simulink model "rendezvous_optimization_ALO"  (R2023a)
settings: Solver=VariableStepAuto  StartTime=0.0  StopTime=600  RelTol=1e-3
undefined symbols (not defined in the file): Ax, Ax_i, Ay, Ay_i, Az, Bx, Bx_i, By, By_i, Bz, Cx, Cx_i, Cy, Cy_i, Cz, IC_x_init, IC_y_init, juliandate, m0, mDot, OC_x_init, OC_y_init, OC_z_init, omega_T, Ve
(part 2 of 2)

== matlab function rendezvous_optimization_ALO/Deputy Spacecraft/Guidance and Control/Control/Translational Controller/MATLAB Function3 ==
  data: rc_N input; Fb_Hill output; vc_N input; Fb_ICRF input
function Fb_Hill = convertForceICRFtoHill(rc_N, vc_N, Fb_ICRF)
%#codegen
% Converts a force vector from ICRF frame to Hill frame
%
% Inputs:
%   rc_N     - Chief inertial position (3x1)
%   vc_N     - Chief inertial velocity (3x1)
%   Fb_ICRF  - Force vector in ICRF frame (3x1)
%
% Output:
%   Fb_Hill  - Force vector in Hill frame (3x1)

% Normalize radial (x) direction
ir = rc_N / norm(rc_N);

% Compute angular momentum vector and normalize (z-direction)
h = cross(rc_N, vc_N);
ih = h / norm(h);

% Compute along-track (y) direction
itheta = cross(ih, ir);

% Construct rotation matrix: Hill to ICRF
R_hill_to_icrf = [ir, itheta, ih];

% To convert from ICRF to Hill: transpose (inverse of rotation matrix)
R_icrf_to_hill = R_hill_to_icrf';

% Rotate force vector into Hill frame
Fb_Hill = R_icrf_to_hill * Fb_ICRF;

end

== matlab function rendezvous_optimization_ALO/Deputy Spacecraft/Guidance and Control/Control/Translational Controller/Outer Controller-x/Controller-1/MATLAB Function ==
  settings: updateMethod=DISCRETE
  data: bestKi output; bestKp output; bestKd output; error input
function [bestKi,bestKp,bestKd] = antlion(error)
% antlion  Tune PID gains [Kp,Ki,Kd] via Ant Lion Optimizer
%
%   sys  = your state‐space or transfer‐function plant
%   [bestKp,bestKi,bestKd] = antlion(sys)

  %% ALO parameters
  nAnt     = 20;          
  Max_iter = 100;
  dim = 3;
  lb       = [0   0   0];  
  ub       = [30 20 30];  

  %% Run Ant Lion Optimizer
  %bestGains = runALO(error, nAnt, Max_iter, lb, ub);
  %bestKp = bestGains(1);
  %bestKi = bestGains(2);
  %bestKd = bestGains(3);
  %fprintf('Optimized gains: Kp=%.4f, Ki=%.4f, Kd=%.4f\n', ...
  %        bestKp, bestKi, bestKd);

   % Initialization
  antlions = rand(nAnt,dim) .* (ub - lb) + lb;
  ants     = zeros(nAnt, dim);
  fitAL    = inf(nAnt,1);
  
  % Evaluate initial fitness
  for i = 1:nAnt
      fitAL(i) = error;
  end
  elite = antlions(1,:);  % Initial elite antlion
  bestScore = fitAL(1);
  % Main loop
  for iter = 1:Max_iter
      % Update elite antlion
      [currBest, idx] = min(fitAL);
      if currBest < bestScore
          elite = antlions(idx,:);
          bestScore = currBest;
      end
      % Adaptive narrowing boundaries
      I = 10^iter/Max_iter;
      for i = 1:nAnt
          % Roulette wheel selection
          selectedAL = antlions(RouletteWheelSelection(1./(fitAL + eps)), :);
          % Random walk around selectedAL and elite
          RW1 = createRandomWalk(iter, Max_iter, lb, ub);
          RW2 = createRandomWalk(iter, Max_iter, lb, ub);
          ants(i,:) = (RW1 + RW2) / 2;
          % Bounds check
          ants(i,:) = max(min(ants(i,:), ub), lb);
      end
      % Evaluate ants
      fitAnts = inf(nAnt,1);
      for i = 1:nAnt
          fitAnts(i) = error;
      end
      % Merge and select next gen
      allPop = [antlions; ants];
      allFit = [fitAL; fitAnts];
      [allFit, idx] = sort(allFit);
      antlions = allPop(idx(1:nAnt), :);
      fitAL    = allFit(1:nAnt);
  end
  bestKp = elite(1); bestKi = elite(2); bestKd = elite(3);
end

%% Helper: Random walk (normalized)
function RW = createRandomWalk(iter, Max_iter, lb, ub)
    steps = 2*(rand(1,Max_iter)>0.5) - 1;
    walk = cumsum(steps);
    walk = (walk - min(walk)) / max(1e-6, max(walk) - min(walk)); % normalized
    RW = lb + walk(iter) .* (ub - lb);
end

%% Helper: Roulette Wheel
function idx = RouletteWheelSelection(probabilities)
    C = cumsum(probabilities / sum(probabilities));
    r = rand;
    idx = find(C >= r, 1, 'first');
end



%function bestGains = runALO(error, nAnt, Max_iter, lb, ub)
%  dim      = numel(lb);
%  antlions = rand(nAnt,dim).*(ub-lb)+lb;
%  ants      = zeros(nAnt,dim);
%  fitAL     = zeros(nAnt,1);
%
%  % Evaluate initial fitness
%  for i=1:nAnt
%    fitAL(i) = error;
%  end
%
%  for iter=1:Max_iter
%    % Roulette wheel selection
%    invFit = 1./(fitAL+eps);
%    P      = invFit/sum(invFit);
%    C      = cumsum(P);
%
%    % Move ants
%    for i=1:nAnt
%      r   = rand;
%      sel = find(C>=r,1);
%      AL  = antlions(sel,:);    % 1×3
%
%      RW = zeros(1,dim);
%      for d=1:dim
%        RW(d) = randomWalk(iter,Max_iter, lb(d), ub(d));
%      end
%
%      ants(i,:) = max(min(AL+RW, ub), lb);
%    end
%
%    % Evaluate ants
%    fitAnts = zeros(nAnt,1);
%    for i=1:nAnt
%      fitAnts(i) = error;
%    end
%
%    % Combine and select next generation antlions
%    allPop   = [antlions; ants];
%    allFit   = [fitAL; fitAnts];
%    [allFit, idx] = sort(allFit);
%    antlions = allPop(idx(1:nAnt), :);
%    fitAL    = allFit(1:nAnt);
%  end
%
%  bestGains = antlions(1,:);
%end
%
%
%function val = randomWalk(iter, Max_iter, lb, ub)
%  steps = 2*(rand(1,Max_iter)>0.5)-1;
%  walk  = cumsum(steps);
%  mn    = min(walk); mx = max(walk);
%  if mx>mn
%    normWalk = (walk-mn)/(mx-mn);
%  else
%    normWalk = zeros(size(walk));
%  end
%  val = lb + normWalk(iter)*(ub-lb);
%end

== matlab function rendezvous_optimization_ALO/Deputy Spacecraft/Guidance and Control/Control/Translational Controller/Outer Controller-z/Controller-3/MATLAB Function ==
  settings: updateMethod=DISCRETE
  data: bestKi output; bestKp output; bestKd output; error input
function [bestKi,bestKp,bestKd] = antlion(error)
% antlion  Tune PID gains [Kp,Ki,Kd] via Ant Lion Optimizer
%
%   sys  = your state‐space or transfer‐function plant
%   [bestKp,bestKi,bestKd] = antlion(sys)

  %% ALO parameters
  nAnt     = 20;          
  Max_iter = 100;
  dim = 3;
  lb       = [0   0   0];  
  ub       = [30 20 30];  

  %% Run Ant Lion Optimizer
  %bestGains = runALO(error, nAnt, Max_iter, lb, ub);
  %bestKp = bestGains(1);
  %bestKi = bestGains(2);
  %bestKd = bestGains(3);
  %fprintf('Optimized gains: Kp=%.4f, Ki=%.4f, Kd=%.4f\n', ...
  %        bestKp, bestKi, bestKd);

   % Initialization
  antlions = rand(nAnt,dim) .* (ub - lb) + lb;
  ants     = zeros(nAnt, dim);
  fitAL    = inf(nAnt,1);
  
  % Evaluate initial fitness
  for i = 1:nAnt
      fitAL(i) = error;
  end
  elite = antlions(1,:);  % Initial elite antlion
  bestScore = fitAL(1);
  % Main loop
  for iter = 1:Max_iter
      % Update elite antlion
      [currBest, idx] = min(fitAL);
      if currBest < bestScore
          elite = antlions(idx,:);
          bestScore = currBest;
      end
      % Adaptive narrowing boundaries
      I = 10^iter/Max_iter;
      for i = 1:nAnt
          % Roulette wheel selection
          selectedAL = antlions(RouletteWheelSelection(1./(fitAL + eps)), :);
          % Random walk around selectedAL and elite
          RW1 = createRandomWalk(iter, Max_iter, lb, ub);
          RW2 = createRandomWalk(iter, Max_iter, lb, ub);
          ants(i,:) = (RW1 + RW2) / 2;
          % Bounds check
          ants(i,:) = max(min(ants(i,:), ub), lb);
      end
      % Evaluate ants
      fitAnts = inf(nAnt,1);
      for i = 1:nAnt
          fitAnts(i) = error;
      end
      % Merge and select next gen
      allPop = [antlions; ants];
      allFit = [fitAL; fitAnts];
      [allFit, idx] = sort(allFit);
      antlions = allPop(idx(1:nAnt), :);
      fitAL    = allFit(1:nAnt);
  end
  bestKp = elite(1); bestKi = elite(2); bestKd = elite(3);
end

%% Helper: Random walk (normalized)
function RW = createRandomWalk(iter, Max_iter, lb, ub)
    steps = 2*(rand(1,Max_iter)>0.5) - 1;
    walk = cumsum(steps);
    walk = (walk - min(walk)) / max(1e-6, max(walk) - min(walk)); % normalized
    RW = lb + walk(iter) .* (ub - lb);
end

%% Helper: Roulette Wheel
function idx = RouletteWheelSelection(probabilities)
    C = cumsum(probabilities / sum(probabilities));
    r = rand;
    idx = find(C >= r, 1, 'first');
end



%function bestGains = runALO(error, nAnt, Max_iter, lb, ub)
%  dim      = numel(lb);
%  antlions = rand(nAnt,dim).*(ub-lb)+lb;
%  ants      = zeros(nAnt,dim);
%  fitAL     = zeros(nAnt,1);
%
%  % Evaluate initial fitness
%  for i=1:nAnt
%    fitAL(i) = error;
%  end
%
%  for iter=1:Max_iter
%    % Roulette wheel selection
%    invFit = 1./(fitAL+eps);
%    P      = invFit/sum(invFit);
%    C      = cumsum(P);
%
%    % Move ants
%    for i=1:nAnt
%      r   = rand;
%      sel = find(C>=r,1);
%      AL  = antlions(sel,:);    % 1×3
%
%      RW = zeros(1,dim);
%      for d=1:dim
%        RW(d) = randomWalk(iter,Max_iter, lb(d), ub(d));
%      end
%
%      ants(i,:) = max(min(AL+RW, ub), lb);
%    end
%
%    % Evaluate ants
%    fitAnts = zeros(nAnt,1);
%    for i=1:nAnt
%      fitAnts(i) = error;
%    end
%
%    % Combine and select next generation antlions
%    allPop   = [antlions; ants];
%    allFit   = [fitAL; fitAnts];
%    [allFit, idx] = sort(allFit);
%    antlions = allPop(idx(1:nAnt), :);
%    fitAL    = allFit(1:nAnt);
%  end
%
%  bestGains = antlions(1,:);
%end
%
%
%function val = randomWalk(iter, Max_iter, lb, ub)
%  steps = 2*(rand(1,Max_iter)>0.5)-1;
%  walk  = cumsum(steps);
%  mn    = min(walk); mx = max(walk);
%  if mx>mn
%    normWalk = (walk-mn)/(mx-mn);
%  else
%    normWalk = zeros(size(walk));
%  end
%  val = lb + normWalk(iter)*(ub-lb);
%end

== matlab function rendezvous_optimization_ALO/Deputy Spacecraft/Guidance and Control/Control/Translational Controller/Inner Controller-x/Subsystem/MATLAB Function ==
  settings: updateMethod=DISCRETE
  data: bestKi output; bestKp output; bestKd output; error input
function [bestKi,bestKp,bestKd] = antlion(error)
% antlion  Tune PID gains [Kp,Ki,Kd] via Ant Lion Optimizer
%
%   sys  = your state‐space or transfer‐function plant
%   [bestKp,bestKi,bestKd] = antlion(sys)

  %% ALO parameters
  nAnt     = 20;          
  Max_iter = 100;
  dim = 3;
  lb       = [0   0   0];  
  ub       = [10 5 10];  

  %% Run Ant Lion Optimizer
  %bestGains = runALO(error, nAnt, Max_iter, lb, ub);
  %bestKp = bestGains(1);
  %bestKi = bestGains(2);
  %bestKd = bestGains(3);
  %fprintf('Optimized gains: Kp=%.4f, Ki=%.4f, Kd=%.4f\n', ...
  %        bestKp, bestKi, bestKd);

   % Initialization
  antlions = rand(nAnt,dim) .* (ub - lb) + lb;
  ants     = zeros(nAnt, dim);
  fitAL    = inf(nAnt,1);
  
  % Evaluate initial fitness
  for i = 1:nAnt
      fitAL(i) = error;
  end
  elite = antlions(1,:);  % Initial elite antlion
  bestScore = fitAL(1);
  % Main loop
  for iter = 1:Max_iter
      % Update elite antlion
      [currBest, idx] = min(fitAL);
      if currBest < bestScore
          elite = antlions(idx,:);
          bestScore = currBest;
      end
      % Adaptive narrowing boundaries
      I = 10^iter/Max_iter;
      for i = 1:nAnt
          % Roulette wheel selection
          selectedAL = antlions(RouletteWheelSelection(1./(fitAL + eps)), :);
          % Random walk around selectedAL and elite
          RW1 = createRandomWalk(iter, Max_iter, lb, ub);
          RW2 = createRandomWalk(iter, Max_iter, lb, ub);
          ants(i,:) = (RW1 + RW2) / 2;
          % Bounds check
          ants(i,:) = max(min(ants(i,:), ub), lb);
      end
      % Evaluate ants
      fitAnts = inf(nAnt,1);
      for i = 1:nAnt
          fitAnts(i) = error;
      end
      % Merge and select next gen
      allPop = [antlions; ants];
      allFit = [fitAL; fitAnts];
      [allFit, idx] = sort(allFit);
      antlions = allPop(idx(1:nAnt), :);
      fitAL    = allFit(1:nAnt);
  end
  bestKp = elite(1); bestKi = elite(2); bestKd = elite(3);
end

%% Helper: Random walk (normalized)
function RW = createRandomWalk(iter, Max_iter, lb, ub)
    steps = 2*(rand(1,Max_iter)>0.5) - 1;
    walk = cumsum(steps);
    walk = (walk - min(walk)) / max(1e-6, max(walk) - min(walk)); % normalized
    RW = lb + walk(iter) .* (ub - lb);
end

%% Helper: Roulette Wheel
function idx = RouletteWheelSelection(probabilities)
    C = cumsum(probabilities / sum(probabilities));
    r = rand;
    idx = find(C >= r, 1, 'first');
end



%function bestGains = runALO(error, nAnt, Max_iter, lb, ub)
%  dim      = numel(lb);
%  antlions = rand(nAnt,dim).*(ub-lb)+lb;
%  ants      = zeros(nAnt,dim);
%  fitAL     = zeros(nAnt,1);
%
%  % Evaluate initial fitness
%  for i=1:nAnt
%    fitAL(i) = error;
%  end
%
%  for iter=1:Max_iter
%    % Roulette wheel selection
%    invFit = 1./(fitAL+eps);
%    P      = invFit/sum(invFit);
%    C      = cumsum(P);
%
%    % Move ants
%    for i=1:nAnt
%      r   = rand;
%      sel = find(C>=r,1);
%      AL  = antlions(sel,:);    % 1×3
%
%      RW = zeros(1,dim);
%      for d=1:dim
%        RW(d) = randomWalk(iter,Max_iter, lb(d), ub(d));
%      end
%
%      ants(i,:) = max(min(AL+RW, ub), lb);
%    end
%
%    % Evaluate ants
%    fitAnts = zeros(nAnt,1);
%    for i=1:nAnt
%      fitAnts(i) = error;
%    end
%
%    % Combine and select next generation antlions
%    allPop   = [antlions; ants];
%    allFit   = [fitAL; fitAnts];
%    [allFit, idx] = sort(allFit);
%    antlions = allPop(idx(1:nAnt), :);
%    fitAL    = allFit(1:nAnt);
%  end
%
%  bestGains = antlions(1,:);
%end
%
%
%function val = randomWalk(iter, Max_iter, lb, ub)
%  steps = 2*(rand(1,Max_iter)>0.5)-1;
%  walk  = cumsum(steps);
%  mn    = min(walk); mx = max(walk);
%  if mx>mn
%    normWalk = (walk-mn)/(mx-mn);
%  else
%    normWalk = zeros(size(walk));
%  end
%  val = lb + normWalk(iter)*(ub-lb);
%end

== matlab function rendezvous_optimization_ALO/Deputy Spacecraft/Guidance and Control/Control/Translational Controller/Outer Controller-x/Controller-1/MATLAB Function1 ==
  settings: updateMethod=DISCRETE
  data: reset input; error_percent output; error input
function error_percent = computeScheduledGain(reset,error)
% Compute gain based on percentage error using 1D look-up style logic
%
% Inputs:
%   r_des     : 3x1 desired position vector
%   r_current : 3x1 current position vector (from chaser)
%   r_init    : 3x1 initial position vector
%
% Output:
%   gain      : scalar scheduled gain

    persistent max_error;

    if reset || isempty(max_error)
        max_error = norm(error);  % store initial max error
    end
    
    e_now = norm(error);       % current error
    error_percent = (e_now / max_error)*100;       % normalized error: [0, 1]

   
end
